simulink model "untitled"  (R2024a)
settings: Solver=VariableStepAuto  StartTime=0.0  StopTime=10.0  RelTol=1e-3
values from neighbouring files (symbols this model uses):
  map = csvread(map_csv)    [Dstar_original.m]
settings Model: Creator=l  LastModifiedBy=l

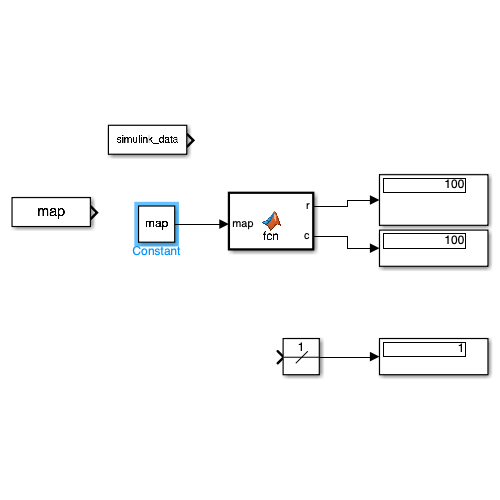
[thumbnail: Simulink's stored preview of the top-level diagram]
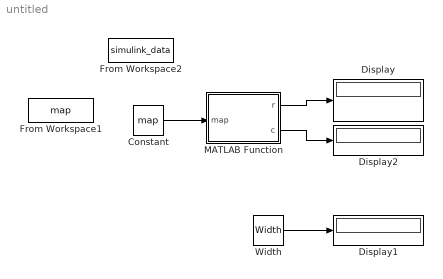
== system untitled ==
  Constant : Constant  Value=map
  Display : Display
  Display1 : Display
  Display2 : Display
  From Workspace1 : FromWorkspace  VariableName=map
  From Workspace2 : FromWorkspace  VariableName=simulink_data
  MATLAB Function : MATLAB Function  TreatAsAtomicUnit=on
  Width : Width
  wires:
  Width/1 -> Display1/1
  MATLAB Function/1(r) -> Display/1
  MATLAB Function/2(c) -> Display2/1
  Constant/1 -> MATLAB Function/1(map)

== matlab function untitled/MATLAB Function ==
  data: map input; r output; c output
function [r,c] = fcn(map)
    % map_data = ones(100,100);
    % [r,c] = size(map_data);
    [r,c] = size(map);
end
